simulink model "PIUIOModelZWSin"  (R2016a)
settings: Solver=VariableStepAuto  StartTime=0.0  StopTime=tEnd  RelTol=1e-3
values from neighbouring files (symbols this model uses):
  A = [-1 1 1;1 -2 0;0 1 -3]    [ExampleActuator.m]    (also in ExampleActuatorSensor.m; ExamplePIUIO.m = [-2 0 1;0 -1 1;1 2 -3]; SinousidPIUIO.m; Untitled.m)
  B = [1;1;0]    [ExampleActuator.m]    (also in ExampleActuatorSensor.m; ExamplePIUIO.m = [1;0;1]; SinousidPIUIO.m; Untitled.m)
  C = [1 0 1;0 1 0]    [ExampleActuator.m]    (also in ExampleActuatorSensor.m; ExamplePIUIO.m = [1 2 3;0 1 2]; SinousidPIUIO.m; Untitled.m)
  d = dTS.Values.Data    [ExampleActuator.m]    (also in ExamplePIUIO.m; SinousidPIUIO.m = 1)
  Ea = [1;0;1]    [ExampleActuatorSensor.m]    (also in ExamplePIUIO.m; SinousidPIUIO.m = [1;0;0]; Untitled.m)
  Ed = [1;0;0]    [ExampleActuator.m]    (also in ExamplePIUIO.m = [1;1;0]; SinousidPIUIO.m = [1;0;1])
  F = A1 - G1*C    [ExampleActuator.m]    (also in ExampleActuatorSensor.m = A1 - G1*Caug; ExamplePIUIO.m = A1-G1*C; SinousidPIUIO.m = A1-G1*C; Untitled.m = A1 - G1*Caug)
  fa_amp = 50    [SinousidPIUIO.m]
  fa_freq = 1    [SinousidPIUIO.m]
  fahat0 = [5]    [ExamplePIUIO.m]    (also in SinousidPIUIO.m = [1])
  G = G1 + A1*N - G1*C*N    [ExampleActuator.m]    (also in ExampleActuatorSensor.m = G1 + A1*N - G1*Caug*N; ExamplePIUIO.m = G1+G2; SinousidPIUIO.m = G1+G2; Untitled.m = G1 + A1*N - G1*Caug*N)
  G1 = P\Y    [ExampleActuator.m]    (also in ExampleActuatorSensor.m; ExamplePIUIO.m = Lhat(1:n,:); SinousidPIUIO.m = Lhat(1:n,:); Untitled.m)
  H = T*B    [ExampleActuator.m]    (also in ExampleActuatorSensor.m = T*Baug; ExamplePIUIO.m; SinousidPIUIO.m; Untitled.m = T*Baug)
  J = T*Ea    [ExamplePIUIO.m]    (also in SinousidPIUIO.m)
  L = Lhat(n+1:end,:)    [ExamplePIUIO.m]    (also in SinousidPIUIO.m)
  M1 = -L*C    [ExamplePIUIO.m]    (also in SinousidPIUIO.m)
  M2 = L*(eye(p)-C*N)    [ExamplePIUIO.m]    (also in SinousidPIUIO.m)
  N = Ed* pinv(C*Ed)    [ExampleActuator.m]    (also in ExampleActuatorSensor.m = Eaug* pinv(Caug*Eaug); ExamplePIUIO.m; SinousidPIUIO.m; Untitled.m = Eaug* pinv(Caug*Eaug))
  R = 0    [ExamplePIUIO.m]    (also in SinousidPIUIO.m = -3)
  w0 = [1;1]    [ExamplePIUIO.m]    (also in SinousidPIUIO.m)
  x0 = [1;2;3]    [ExampleActuator.m]    (also in ExampleActuatorSensor.m; ExamplePIUIO.m; SinousidPIUIO.m; Untitled.m)
  xhat0 = [2;1;1]    [ExamplePIUIO.m]    (also in SinousidPIUIO.m)
  z0 = [0.1;0.2;0.3]    [ExampleActuator.m]    (also in ExampleActuatorSensor.m = [0.1;.2;.3;0.4;0.5]; ExamplePIUIO.m = xhat0; SinousidPIUIO.m = xhat0; Untitled.m = [0.1;0.2;0.3;0.4;0.5])
settings Model: Creator=amirreza513  LastModifiedBy=amirreza513

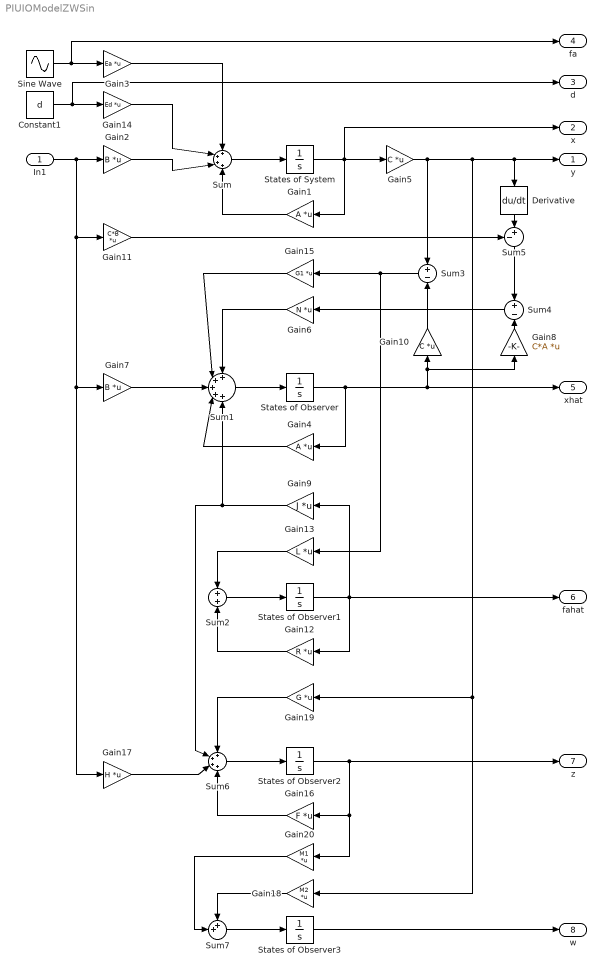
== system PIUIOModelZWSin ==
  In1 : Inport
  Constant1 : Constant  Value=d
  Derivative : Derivative  CoefficientInTFapproximation=0
  Gain1 : Gain  Gain=A  Multiplication=Matrix(K*u) (u vector)
  Gain10 : Gain  Gain=C  Multiplication=Matrix(K*u) (u vector)
  Gain11 : Gain  Gain=C*B  Multiplication=Matrix(K*u) (u vector)
  Gain12 : Gain  Gain=R  Multiplication=Matrix(K*u) (u vector)
  Gain13 : Gain  Gain=L  Multiplication=Matrix(K*u) (u vector)
  Gain14 : Gain  Gain=Ed  Multiplication=Matrix(K*u) (u vector)
  Gain15 : Gain  Gain=G1  Multiplication=Matrix(K*u) (u vector)
  Gain16 : Gain  Gain=F  Multiplication=Matrix(K*u) (u vector)
  Gain17 : Gain  Gain=H  Multiplication=Matrix(K*u) (u vector)
  Gain18 : Gain  Gain=M2  Multiplication=Matrix(K*u) (u vector)
  Gain19 : Gain  Gain=G  Multiplication=Matrix(K*u) (u vector)
  Gain2 : Gain  Gain=B  Multiplication=Matrix(K*u) (u vector)
  Gain20 : Gain  Gain=M1  Multiplication=Matrix(K*u) (u vector)
  Gain3 : Gain  Gain=Ea  Multiplication=Matrix(K*u) (u vector)
  Gain4 : Gain  Gain=A  Multiplication=Matrix(K*u) (u vector)
  Gain5 : Gain  Gain=C  Multiplication=Matrix(K*u) (u vector)
  Gain6 : Gain  Gain=N  Multiplication=Matrix(K*u) (u vector)
  Gain7 : Gain  Gain=B  Multiplication=Matrix(K*u) (u vector)
  Gain8 : Gain  Gain=C*A  Multiplication=Matrix(K*u) (u vector)
  Gain9 : Gain  Gain=J  Multiplication=Matrix(K*u) (u vector)
  Sine Wave : Sin  Amplitude=fa_amp  Frequency=fa_freq  SampleTime=0
  States of Observer : Integrator  InitialCondition=xhat0
  States of Observer1 : Integrator  InitialCondition=fahat0
  States of Observer2 : Integrator  InitialCondition=z0
  States of Observer3 : Integrator  InitialCondition=w0
  States of System : Integrator  InitialCondition=x0
  Sum : Sum  Inputs=++++
  Sum1 : Sum  Inputs=+++++
  Sum2 : Sum
  Sum3 : Sum  Inputs=+-
  Sum4 : Sum  Inputs=+-
  Sum5 : Sum  Inputs=-+|
  Sum6 : Sum  Inputs=++++
  Sum7 : Sum  Inputs=++|
  y : Outport
  x : Outport  Port=2
  d : Outport  Port=3
  fa : Outport  Port=4
  xhat : Outport  Port=5
  fahat : Outport  Port=6
  z : Outport  Port=7
  w : Outport  Port=8
  wires:
  States of System/1 -> x/1, Gain5/1, Gain1/1
  In1/1 -> Gain17/1, Gain7/1, Gain11/1, Gain2/1
  Sine Wave/1 -> fa/1, Gain3/1
  Sum/1 -> States of System/1
  Gain5/1 -> Sum3/1, Gain18/1, Gain19/1, Derivative/1, y/1
  Gain3/1 -> Sum/1
  Sum1/1 -> States of Observer/1
  States of Observer/1 -> xhat/1, Gain8/1, Gain10/1, Gain4/1
  Constant1/1 -> Gain14/1, d/1
  Gain14/1 -> Sum/2
  Gain2/1 -> Sum/3
  Gain1/1 -> Sum/4
  Gain7/1 -> Sum1/3
  Gain4/1 -> Sum1/4
  Sum3/1 -> Gain13/1, Gain15/1
  Gain10/1 -> Sum3/2
  Gain15/1 -> Sum1/2
  Gain6/1 -> Sum1/1
  Sum4/1 -> Gain6/1
  Gain8/1 -> Sum4/2
  Derivative/1 -> Sum5/2
  Gain11/1 -> Sum5/1
  Sum5/1 -> Sum4/1
  Gain9/1 -> Sum6/2, Sum1/5
  States of Observer1/1 -> Gain9/1, Gain12/1, fahat/1
  Sum2/1 -> States of Observer1/1
  Gain12/1 -> Sum2/2
  Gain13/1 -> Sum2/1
  States of Observer2/1 -> z/1, Gain20/1, Gain16/1
  Sum6/1 -> States of Observer2/1
  Gain16/1 -> Sum6/4
  Gain17/1 -> Sum6/3
  Gain19/1 -> Sum6/1
  States of Observer3/1 -> w/1
  Sum7/1 -> States of Observer3/1
  Gain18/1 -> Sum7/1
  Gain20/1 -> Sum7/2
